simulink model "grid_converter_power_control"  (R2024b)
settings: Solver=ode45  StartTime=0  StopTime=.1  MaxStep=T_s  RelTol=1e-3  AbsTol=1e-3  EnableMultiTasking=on
values from neighbouring files (symbols this model uses):
  alpha_c = 2*pi*400    (= 2513.27412287)    [init.m]    (also in init_vector.m = 3769.91118431)
  L_f = 10e-3    (= 0.01)    [init.m]
  T_s = 1/(2*f_sw)    (= 6.25e-05)    [init.m]    (also in init_vector.m = 0.000125; init_vhz.m = 0.000125)
  u_gN = sqrt(2/3)*400    [init.m]
  w0_pll = 2*pi*20    (= 125.663706144)    [init.m]
  w_g = 2*pi*50    (= 314.159265359)    [init.m]
libraries: simulink x1
settings Model: Creator=mhinkkan  LastModifiedBy=Admin
settings SolverCC: AutoScaleAbsTol=off  AlgebraicLoopSolver=TrustRegion
settings DataIOCC: SaveFormat=Array  SignalLoggingSaveFormat=ModelDataLogs  SaveOutput=off  SignalLogging=off  DSMLogging=off  SaveTime=off  ReturnWorkspaceOutputs=off
settings OptimizationCC: BlockReduction=off  BooleanDataType=off  DefaultParameterBehavior=Inlined  OptimizeBlockIOStorage=off  BufferReuse=off  ReuseModelBlockBuffer=off  ExpressionFolding=off  ExpressionDepthLimit=2147483647  LocalBlockOutputs=off  InitFltsAndDblsToZero=on  LifeSpan=inf
settings DebuggingCC: SaveWithParameterizedLinksMsg=none  UnderspecifiedInitializationDetection=Classic  MergeDetectMultiDrivingBlocksExec=none  SignalResolutionControl=TryResolveAllWithWarning  MultiTaskDSMMsg=warning  MultiTaskCondExecSysMsg=none  FcnCallInpInsideContextMsg=warning  UnconnectedInputMsg=warning  UnconnectedOutputMsg=warning  UnconnectedLineMsg=warning  StateNameClashWarn=warning  SFUnexpectedBacktrackingDiag=warning  SFNoUnconditionalDefaultTransitionDiag=warning  SFExecutionAtInitializationDiag=none  ArithmeticOperatorsInVariantConditions=warning
settings HardwareCC: ProdBitPerPointer=32  ProdBitPerSizeT=32  ProdBitPerPtrDiffT=32  ProdLargestAtomicFloat=None  ProdIntDivRoundTo=Undefined  ProdEndianess=Unspecified  ProdWordSize=32  ProdHWDeviceType=32-bit Generic  TargetUnknown=on
settings ModelReferenceCC: PropagateSignalLabelsOutOfModel=off
settings SFSimCC: SimUseLocalCustomCode=off  CustomCodeUndefinedFunction=UseInterfaceOnly
settings RTWCC: RTWUseLocalCustomCode=off  GPUComputeCapability=3.5
settings CodeAppCC: StateflowObjectComments=on
settings GRTTargetCC: TargetFcnLib=ansi_tfl_tmw.mat  TargetLangStandard=C89/C90 (ANSI)  CombineOutputUpdateFcns=off  GRTInterface=on
settings ConfigComp: CovMetricSettings=dw  CovSaveCumulativeToWorkspaceVar=on  CovSaveSingleToWorkspaceVar=on  CovExternalEMLEnable=off

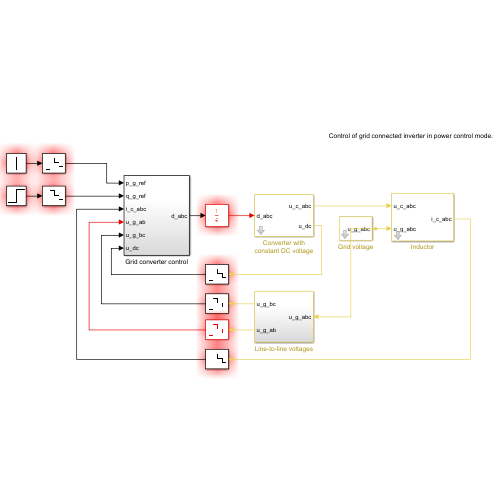
[thumbnail: Simulink's stored preview of the top-level diagram]
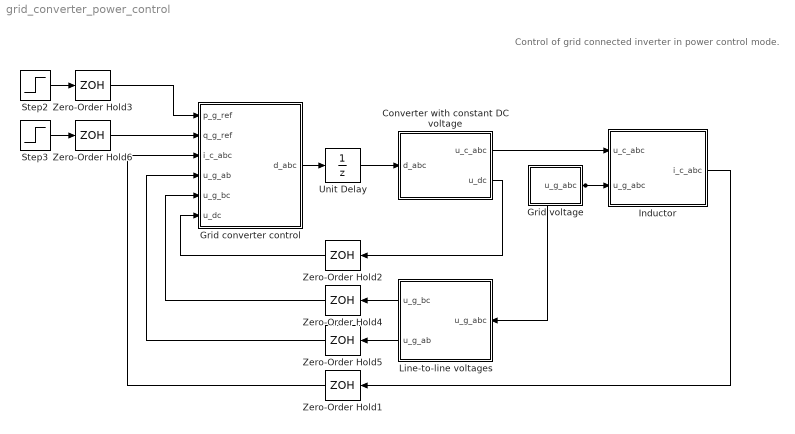
== system grid_converter_power_control ==
  note: Control of grid connected inverter in power control mode.
  "Converter with constant DC voltage " : Subsystem  mask{f_sw=8e3, u_dc=650}
      mask prompts: f_sw "Switching frequency (Hz)"; u_dc "DC-bus voltage (V)"
      mask init:
      | T_s = 1/(2*f_sw);
  Grid converter control : Subsystem
  Grid voltage : Subsystem  mask{w_g=2*pi*50, U_g=400}
      mask prompts: w_g "Grid angular frequency (rad/s)"; U_g "Line-line rms grid voltage (V)"
  Inductor : Subsystem  mask{L_f=10e-3, R_f=0}
      mask prompts: L_f "Inductance (H)"; R_f "Series resistance (ohm)"
  Line-to-line voltages : Subsystem
  Step2 : Step  Time=0.02  After=5e3  SampleTime=T_s
  Step3 : Step  Time=0.04  After=4e3  SampleTime=T_s
  Unit Delay : UnitDelay  SampleTime=T_s  HasFrameUpgradeWarning=on
  Zero-Order Hold{1..6} (6 alike) : ZeroOrderHold  SampleTime=T_s
  wires:
  Zero-Order Hold3/1 -> Grid converter control/1(p_g_ref)
  Zero-Order Hold1/1 -> Grid converter control/3(i_c_abc)
  Zero-Order Hold2/1 -> Grid converter control/6(u_dc)
  Step2/1 -> Zero-Order Hold3/1
  "Converter with constant DC voltage "/1(u_c_abc) -> Inductor/1(u_c_abc)
  Zero-Order Hold4/1 -> Grid converter control/5(u_g_bc)
  Zero-Order Hold5/1 -> Grid converter control/4(u_g_ab)
  Grid converter control/1(d_abc) -> Unit Delay/1
  Step3/1 -> Zero-Order Hold6/1
  Zero-Order Hold6/1 -> Grid converter control/2(q_g_ref)
  "Converter with constant DC voltage "/2(u_dc) -> Zero-Order Hold2/1
  Inductor/1(i_c_abc) -> Zero-Order Hold1/1
  Unit Delay/1 -> "Converter with constant DC voltage "/1(d_abc)
  Grid voltage/1(u_g_abc) -> Line-to-line voltages/1(u_g_abc), Inductor/2(u_g_abc)
  Line-to-line voltages/1(u_g_bc) -> Zero-Order Hold4/1
  Line-to-line voltages/2(u_g_ab) -> Zero-Order Hold5/1

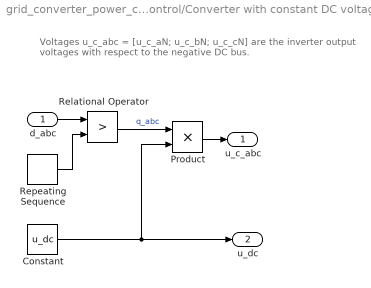
== system grid_converter_power_control/Converter with constant DC voltage  ==
  note: Voltages u_c_abc = [u_c_aN; u_c_bN; u_c_cN] are the inverter
      | output voltages with respect to the negative DC bus.
  d_abc : Inport
  Constant : Constant  Value=u_dc
  Product : Product
  Relational Operator : RelationalOperator  Operator=>  OutDataTypeStr='double'  InputSameDT=off
  Repeating Sequence : simulink/Sources/Repeating Sequence  rep_seq_t=[0 1 2]*T_s  rep_seq_y=[1 0 1]
  u_c_abc : Outport
  u_dc : Outport  Port=2
  wires:
  Repeating Sequence/1 -> Relational Operator/2
  d_abc/1 -> Relational Operator/1
  Product/1 -> u_c_abc/1
  Relational Operator/1 -> Product/1  "q_abc"
  Constant/1 -> Product/2, u_dc/1

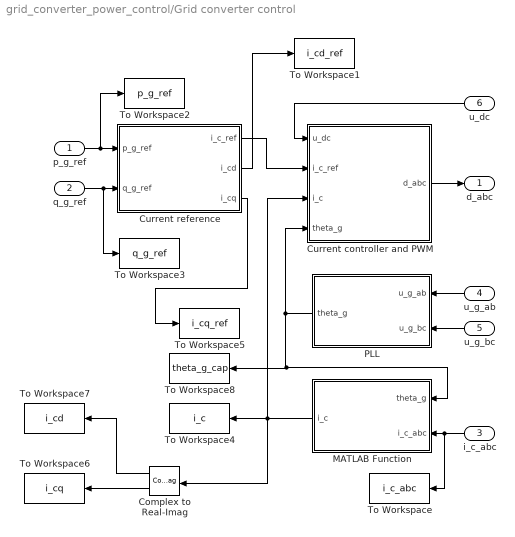
== system grid_converter_power_control/Grid converter control ==
  p_g_ref : Inport
  q_g_ref : Inport  Port=2
  i_c_abc : Inport  Port=3
  u_g_ab : Inport  Port=4
  u_g_bc : Inport  Port=5
  u_dc : Inport  Port=6
  Complex to Real-Imag : ComplexToRealImag
  Current controller and PWM : Subsystem
  Current reference : MATLAB Function  TreatAsAtomicUnit=on
  MATLAB Function : MATLAB Function  TreatAsAtomicUnit=on
  PLL : Subsystem
  To Workspace : ToWorkspace  VariableName=i_c_abc  SaveFormat=Timeseries  SampleTime=-1
  To Workspace1 : ToWorkspace  VariableName=i_cd_ref  SaveFormat=Timeseries  SampleTime=-1
  To Workspace2 : ToWorkspace  VariableName=p_g_ref  SaveFormat=Timeseries  SampleTime=-1
  To Workspace3 : ToWorkspace  VariableName=q_g_ref  SaveFormat=Timeseries  SampleTime=-1
  To Workspace4 : ToWorkspace  VariableName=i_c  SaveFormat=Timeseries  SampleTime=-1
  To Workspace5 : ToWorkspace  VariableName=i_cq_ref  SaveFormat=Timeseries  SampleTime=-1
  To Workspace6 : ToWorkspace  VariableName=i_cq  SaveFormat=Timeseries  SampleTime=-1
  To Workspace7 : ToWorkspace  VariableName=i_cd  SaveFormat=Timeseries  SampleTime=-1
  To Workspace8 : ToWorkspace  VariableName=theta_g_cap  SaveFormat=Timeseries  SampleTime=-1
  d_abc : Outport
  wires:
  i_c_abc/1 -> To Workspace/1, MATLAB Function/2(i_c_abc)
  Current controller and PWM/1(d_abc) -> d_abc/1
  Current reference/1(i_c_ref) -> Current controller and PWM/2(i_c_ref)
  MATLAB Function/1(i_c) -> Complex to Real-Imag/1, To Workspace4/1, Current controller and PWM/3(i_c)
  q_g_ref/1 -> To Workspace3/1, Current reference/2(q_g_ref)
  p_g_ref/1 -> To Workspace2/1, Current reference/1(p_g_ref)
  u_g_bc/1 -> PLL/2(u_g_bc)
  u_g_ab/1 -> PLL/1(u_g_ab)
  PLL/1(theta_g) -> Current controller and PWM/4(theta_g), To Workspace8/1, MATLAB Function/1(theta_g)
  u_dc/1 -> Current controller and PWM/1(u_dc)
  Current reference/2(i_cd) -> To Workspace1/1
  Current reference/3(i_cq) -> To Workspace5/1
  Complex to Real-Imag/2 -> To Workspace6/1
  Complex to Real-Imag/1 -> To Workspace7/1

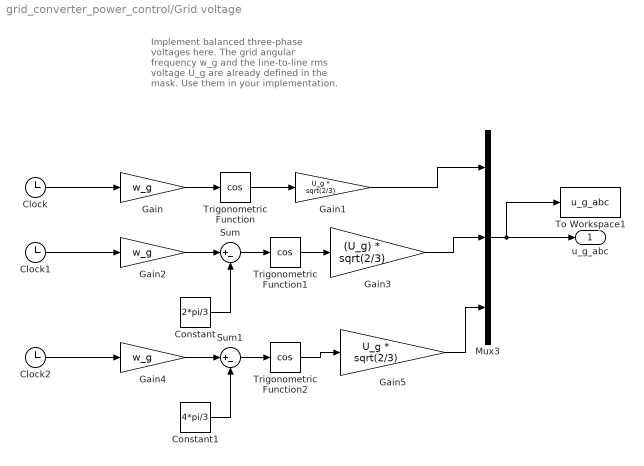
== system grid_converter_power_control/Grid voltage ==
  note: Implement balanced three-phase
      | voltages here. The grid angular
      | frequency w_g and the line-to-line rms
      | voltage U_g are already defined
      | in the mask. Use them in your
      | implementation.
  Clock : Clock
  Clock1 : Clock
  Clock2 : Clock
  Constant : Constant  Value=2*pi/3
  Constant1 : Constant  Value=4*pi/3
  Gain : Gain  Gain=w_g
  Gain1 : Gain  Gain=U_g * sqrt(2/3)
  Gain2 : Gain  Gain=w_g
  Gain3 : Gain  Gain=(U_g) * sqrt(2/3)
  Gain4 : Gain  Gain=w_g
  Gain5 : Gain  Gain=U_g * sqrt(2/3)
  Mux3 : Mux  Inputs=3
  Sum : Sum  Inputs=|+-
  Sum1 : Sum  Inputs=|+-
  To Workspace1 : ToWorkspace  VariableName=u_g_abc  SaveFormat=Timeseries  SampleTime=-1
  Trigonometric Function : Trigonometry  Operator=cos
  Trigonometric Function1 : Trigonometry  Operator=cos
  Trigonometric Function2 : Trigonometry  Operator=cos
  u_g_abc : Outport
  wires:
  Mux3/1 -> To Workspace1/1, u_g_abc/1
  Clock/1 -> Gain/1
  Gain/1 -> Trigonometric Function/1
  Trigonometric Function/1 -> Gain1/1
  Gain1/1 -> Mux3/1
  Trigonometric Function1/1 -> Gain3/1
  Clock1/1 -> Gain2/1
  Gain2/1 -> Sum/1
  Sum/1 -> Trigonometric Function1/1
  Gain3/1 -> Mux3/2
  Constant/1 -> Sum/2
  Constant1/1 -> Sum1/2
  Gain4/1 -> Sum1/1
  Trigonometric Function2/1 -> Gain5/1
  Sum1/1 -> Trigonometric Function2/1
  Clock2/1 -> Gain4/1
  Gain5/1 -> Mux3/3

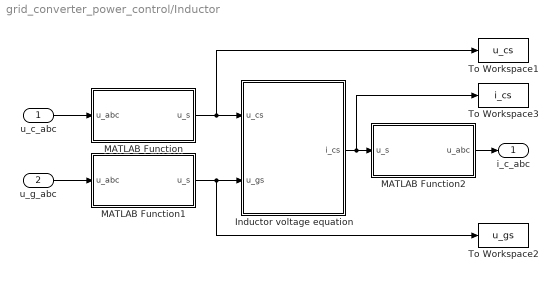
== system grid_converter_power_control/Inductor ==
  u_c_abc : Inport
  u_g_abc : Inport  Port=2
  Inductor voltage equation : Subsystem
  MATLAB Function : MATLAB Function  TreatAsAtomicUnit=on
  MATLAB Function1 : MATLAB Function  TreatAsAtomicUnit=on
  MATLAB Function2 : MATLAB Function  TreatAsAtomicUnit=on
  To Workspace1 : ToWorkspace  VariableName=u_cs  SaveFormat=Timeseries
  To Workspace2 : ToWorkspace  VariableName=u_gs  SaveFormat=Timeseries
  To Workspace3 : ToWorkspace  VariableName=i_cs  SaveFormat=Timeseries
  i_c_abc : Outport
  wires:
  u_c_abc/1 -> MATLAB Function/1(u_abc)
  Inductor voltage equation/1(i_cs) -> To Workspace3/1, MATLAB Function2/1(u_s)
  MATLAB Function/1(u_s) -> Inductor voltage equation/1(u_cs), To Workspace1/1
  MATLAB Function2/1(u_abc) -> i_c_abc/1
  MATLAB Function1/1(u_s) -> To Workspace2/1, Inductor voltage equation/2(u_gs)
  u_g_abc/1 -> MATLAB Function1/1(u_abc)

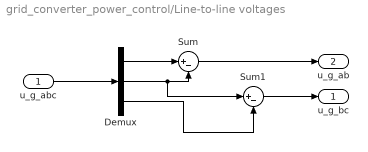
== system grid_converter_power_control/Line-to-line voltages ==
  u_g_abc : Inport
  Demux : Demux  Outputs=3
  Sum : Sum  Inputs=|+-
  Sum1 : Sum  Inputs=|+-
  u_g_bc : Outport
  u_g_ab : Outport  Port=2
  wires:
  u_g_abc/1 -> Demux/1
  Demux/1 -> Sum/1
  Demux/2 -> Sum1/1, Sum/2
  Sum/1 -> u_g_ab/1
  Demux/3 -> Sum1/2
  Sum1/1 -> u_g_bc/1

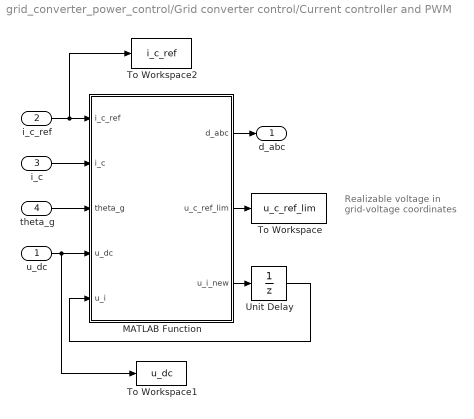
== system grid_converter_power_control/Grid converter control/Current controller and PWM ==
  note: Realizable voltage
      | in grid-voltage coordinates
  u_dc : Inport
  i_c_ref : Inport  Port=2
  i_c : Inport  Port=3
  theta_g : Inport  Port=4
  MATLAB Function : MATLAB Function  TreatAsAtomicUnit=on
  To Workspace : ToWorkspace  VariableName=u_c_ref_lim  SaveFormat=Timeseries  SampleTime=-1
  To Workspace1 : ToWorkspace  VariableName=u_dc  SaveFormat=Timeseries  SampleTime=-1
  To Workspace2 : ToWorkspace  VariableName=i_c_ref  SaveFormat=Timeseries  SampleTime=-1
  Unit Delay : UnitDelay  InitialCondition=u_gN  SampleTime=-1  HasFrameUpgradeWarning=on
  d_abc : Outport  PortDimensions=3
  wires:
  MATLAB Function/3(u_i_new) -> Unit Delay/1
  i_c_ref/1 -> To Workspace2/1, MATLAB Function/1(i_c_ref)
  i_c/1 -> MATLAB Function/2(i_c)
  Unit Delay/1 -> MATLAB Function/5(u_i)
  MATLAB Function/1(d_abc) -> d_abc/1
  MATLAB Function/2(u_c_ref_lim) -> To Workspace/1
  theta_g/1 -> MATLAB Function/3(theta_g)
  u_dc/1 -> To Workspace1/1, MATLAB Function/4(u_dc)

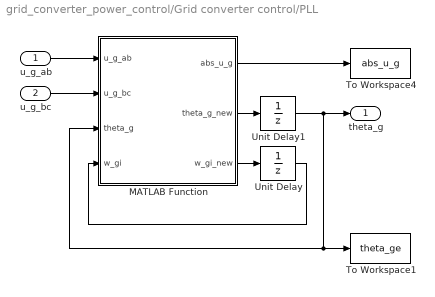
== system grid_converter_power_control/Grid converter control/PLL ==
  u_g_ab : Inport
  u_g_bc : Inport  Port=2
  MATLAB Function : MATLAB Function  TreatAsAtomicUnit=on
  To Workspace1 : ToWorkspace  VariableName=theta_ge  SaveFormat=Timeseries  SampleTime=-1
  To Workspace4 : ToWorkspace  VariableName=abs_u_g  SaveFormat=Timeseries  SampleTime=-1
  Unit Delay : UnitDelay  InitialCondition=w_g  SampleTime=-1  HasFrameUpgradeWarning=on
  Unit Delay1 : UnitDelay  SampleTime=-1  HasFrameUpgradeWarning=on
  theta_g : Outport
  wires:
  u_g_bc/1 -> MATLAB Function/2(u_g_bc)
  u_g_ab/1 -> MATLAB Function/1(u_g_ab)
  MATLAB Function/1(abs_u_g) -> To Workspace4/1
  MATLAB Function/3(w_gi_new) -> Unit Delay/1
  MATLAB Function/2(theta_g_new) -> Unit Delay1/1
  Unit Delay1/1 -> MATLAB Function/3(theta_g), To Workspace1/1, theta_g/1
  Unit Delay/1 -> MATLAB Function/4(w_gi)

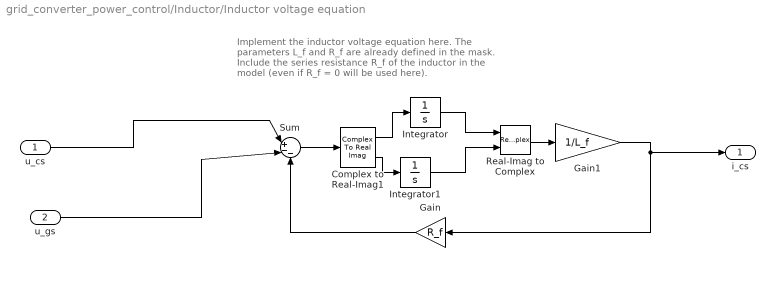
== system grid_converter_power_control/Inductor/Inductor voltage equation ==
  note: Implement the inductor voltage equation here.
      | The parameters L_f and R_f are already defined in the
      | mask. Include the series resistance R_f of the inductor
      | in the model (even if R_f = 0 will be used here).
  u_cs : Inport
  u_gs : Inport  Port=2
  Complex to Real-Imag1 : ComplexToRealImag
  Gain : Gain  Gain=R_f
  Gain1 : Gain  Gain=1/L_f
  Integrator : Integrator
  Integrator1 : Integrator
  Real-Imag to Complex : RealImagToComplex
  Sum : Sum  Inputs=|+--
  i_cs : Outport
  wires:
  u_cs/1 -> Sum/1
  u_gs/1 -> Sum/2
  Sum/1 -> Complex to Real-Imag1/1
  Complex to Real-Imag1/2 -> Integrator1/1
  Complex to Real-Imag1/1 -> Integrator/1
  Integrator/1 -> Real-Imag to Complex/1
  Integrator1/1 -> Real-Imag to Complex/2
  Real-Imag to Complex/1 -> Gain1/1
  Gain1/1 -> Gain/1, i_cs/1
  Gain/1 -> Sum/3

== matlab function grid_converter_power_control/Grid converter control/Current controller and PWM/MATLAB Function ==
  data: i_c_ref input size=1; i_c input size=1; theta_g input size=1; u_dc input size=1; u_i input size=1; w_g parameter size=1; L_f parameter size=1; alpha_c parameter size=1; T_s parameter size=1; d_abc output size=3; u_c_ref_lim output size=1; u_i_new output size=1
function [d_abc, u_c_ref_lim, u_i_new] = cc(i_c_ref, i_c, ...
    theta_g, u_dc, u_i, w_g, L_f, alpha_c, T_s)

%% Current controller 
% Gains
k_i = alpha_c^2*L_f;                % Integral gain
k_t = alpha_c*L_f;                  % Reference gain
k_p = (2*alpha_c - 1j*w_g)*L_f;     % Proportional gain

% Voltage reference in synchronous coordinates
u_c_ref = k_t*i_c_ref - k_p*i_c + u_i;

% Reference in stator coordinates
theta_gc = theta_g + 1.5*T_s*w_g;   % Compensation for discrete-time delays
u_cs_ref = u_c_ref*exp(1j*theta_gc);

%% Symmetrical suboscillation PWM
% Components of the voltage space vector
u_c_alpha_ref = real(u_cs_ref);
u_c_beta_ref  = imag(u_cs_ref);

% Phase-voltage references
u_ca_ref = u_c_alpha_ref;
u_cb_ref = .5*(-u_c_alpha_ref + sqrt(3)*u_c_beta_ref);
u_cc_ref = .5*(-u_c_alpha_ref - sqrt(3)*u_c_beta_ref);

% Vector of phase-voltage references
u_c_abc_ref = [u_ca_ref; u_cb_ref; u_cc_ref];

% Symmetrization of the references by adding the zero-sequence voltage
u0 = .5*(max(u_c_abc_ref) + min(u_c_abc_ref));
u_c_abc_ref = u_c_abc_ref - u0;

% Clipping of the reference voltages such that no phase error is caused. 
% If all phase voltage reference are realizable (below u_dc/2), m = 1 holds.
m = max([2*u_c_abc_ref/u_dc; 1]);
u_c_abc_ref = u_c_abc_ref/m;

% Duty cycles, which can be directly used for triangle comparison, 
% if the triangle wave varies between 0...1
d_abc = .5 + u_c_abc_ref/u_dc;

% Realized voltage vector is calculated from the clamped duty ratios.
% If the PWM does not saturate, u_c_ref_lim = u_c_ref holds. The realized
% voltage vector is needed, e.g., for the current-controller antiwindup.
u_cs_ref_lim = 2/3*(d_abc(1) + d_abc(2)*exp(1j*2*pi/3) ...
    + d_abc(3)*exp(1j*4*pi/3))*u_dc;
% In estimated rotor flux coordinates
u_c_ref_lim = exp(-1j*theta_gc)*u_cs_ref_lim;  

%% Update the integral state of the current controller 
u_i_new = u_i + T_s*k_i*(i_c_ref - i_c + (u_c_ref_lim - u_c_ref)/k_t);

== matlab function grid_converter_power_control/Grid converter control/PLL/MATLAB Function ==
  data: u_g_ab input size=1; u_g_bc input size=1; theta_g input; w_gi input; u_gN parameter; w0_pll parameter; abs_u_g output size=1; theta_g_new output; w_gi_new output; T_s parameter
function [abs_u_g, theta_g_new, w_gi_new] = pll(u_g_ab, u_g_bc, ...
    theta_g, w_gi, u_gN, w0_pll, T_s)

% Parameters 
% (Tuning of the PLL is analogous to that of the DC-voltage controller.)
zeta = 1;   % Damping ratio
k_p = 2*zeta*w0_pll/u_gN; 
k_i = w0_pll^2/u_gN;

% Space-vector transformation from line-to-line components
u_gs = 2/3 *(u_g_ab - u_g_bc*exp(1i *4*pi/3));  % Complete this

% Coordinate transformation to the "estimated" grid coordinates
u_g = u_gs * exp(-theta_g * 1i);  % Complete this

% Error signal, which is drive to zero by the PLL
u_gq = imag(u_g); % Complete this

w_g = k_p*u_gq + w_gi;

% Update the integral state
w_gi_new = w_gi + T_s*k_i*u_gq;

% Update the grid-voltage angle
theta_g_new = theta_g + T_s*w_g;
while(theta_g_new > pi)
    theta_g_new = theta_g_new - 2*pi;
end
while(theta_g_new < -pi)
    theta_g_new = theta_g_new + 2*pi;
end

% Absolute value of the grid-voltage vector
abs_u_g = abs(u_g);

== matlab function grid_converter_power_control/Grid converter control/Current reference ==
  data: p_g_ref input; q_g_ref input; i_c_ref output; u_gN parameter size=1; i_cd output; i_cq output
function [i_c_ref,i_cd, i_cq] = curr_ref(p_g_ref, q_g_ref, u_gN)

% Current references in grid-voltage coordinates
i_cd = 2/3*p_g_ref/u_gN;
i_cq= -2/3*q_g_ref/u_gN;
i_c_ref = i_cd + j*i_cq; % Complete this

== matlab function grid_converter_power_control/Grid converter control/MATLAB Function ==
  data: theta_g input size=1; i_c_abc input size=3; i_c output size=1
function i_c = abc2dq(theta_g, i_c_abc)

% Space-vector transformation
i_cs = 2/3*(i_c_abc(1) + i_c_abc(2)*exp(1j*2*pi/3) ...
    + i_c_abc(3)*exp(1j*4*pi/3));

% Coordinate transformation
i_c = i_cs*exp(-1j*theta_g);

== matlab function grid_converter_power_control/Inductor/MATLAB Function ==
  data: u_abc input size=3; u_s output size=1
function u_s = abc2s(u_abc)

% Space-vector transformation
u_s = 2/3*(u_abc(1) + u_abc(2)*exp(1j*2*pi/3) + u_abc(3)*exp(1j*4*pi/3));

== matlab function grid_converter_power_control/Inductor/MATLAB Function1 ==
  data: u_abc input size=3; u_s output size=1
function u_s = abc2s(u_abc)

% Space-vector transformation
u_s = 2/3*(u_abc(1) + u_abc(2)*exp(1j*2*pi/3) + u_abc(3)*exp(1j*4*pi/3));

== matlab function grid_converter_power_control/Inductor/MATLAB Function2 ==
  data: u_s input size=1; u_abc output size=3
function u_abc = s2abc(u_s)

% Inverse space-vector transformation
u_abc = real([1; exp(-1j*2*pi/3); exp(-1j*4*pi/3)]*u_s);
